simulink model "vdc_dyc_v3"  (R2020a)
settings: Solver=ode4  StartTime=0.0  StopTime=inf  FixedStep=1e-3  RelTol=1e-3
InitFcn:
  | clear mex
values from neighbouring files (symbols this model uses):
  vicrt_inputfile = append(path_send,              '2261_VOLCANO_ramp_RH12002_send_svm.xml')    [select_maneuver_files.m]
undefined symbols (not defined in the file or in its folder): vicrt_initcallback, vicrt_initmexcallback, vicrt_simulationmanager
libraries: simulink x1
(part 1 of 5)
settings Model: Creator=mcava  LastModifiedBy=lucas
settings DataIOCC: LimitDataPoints=on  SaveFormat=Array  ReturnWorkspaceOutputs=off  SignalLoggingName=sigsOut
settings OptimizationCC: ExpressionDepthLimit=2147483647  InitFltsAndDblsToZero=on  LifeSpan=inf
settings DebuggingCC: SignalInfNanChecking=warning  AlgebraicLoopMsg=none  SaveWithParameterizedLinksMsg=none  UnderspecifiedInitializationDetection=Classic  MergeDetectMultiDrivingBlocksExec=none  SignalResolutionControl=TryResolveAllWithWarning  MultiTaskDSMMsg=warning  MultiTaskCondExecSysMsg=none  FcnCallInpInsideContextMsg=warning  StateNameClashWarn=warning  SFUnexpectedBacktrackingDiag=warning  SFNoUnconditionalDefaultTransitionDiag=warning  SFExecutionAtInitializationDiag=none  ArithmeticOperatorsInVariantConditions=warning
settings HardwareCC: ProdBitPerPointer=32  ProdBitPerSizeT=32  ProdBitPerPtrDiffT=32  ProdLargestAtomicFloat=None  ProdIntDivRoundTo=Undefined  ProdEndianess=Unspecified  ProdWordSize=32  ProdHWDeviceType=32-bit Generic  TargetBitPerPointer=64  TargetBitPerSizeT=64  TargetBitPerPtrDiffT=64  TargetLongLongMode=on  TargetIntDivRoundTo=Zero  TargetEndianess=LittleEndian  TargetWordSize=64  TargetHWDeviceType=MATLAB Host  ProdEqTarget=off
settings ModelReferenceCC: PropagateSignalLabelsOutOfModel=off
settings SFSimCC: SimUseLocalCustomCode=off  SimParseCustomCode=off  CustomCodeUndefinedFunction=UseInterfaceOnly
settings RTWCC: RTWVerbose=off  RTWUseLocalCustomCode=off
settings CodeAppCC: GenerateComments=off  SimulinkBlockComments=off
settings GRTTargetCC: TargetFcnLib=ansi_tfl_tmw.mat  TargetLangStandard=C89/C90 (ANSI)  CombineOutputUpdateFcns=off  GRTInterface=on
settings ConfigComp: CovMetricSettings=dw  CovHtmlReporting=on  CovSaveCumulativeToWorkspaceVar=on  CovSaveSingleToWorkspaceVar=on  CovExternalEMLEnable=off

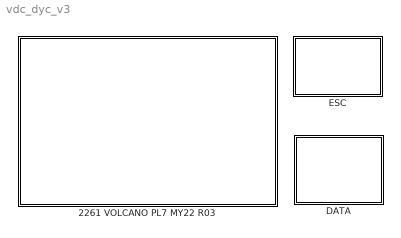
== system vdc_dyc_v3 ==
  2261 VOLCANO PL7 MY22 R03 : Subsystem
      mask Display: image(imread('C:\Users\lucas\Desktop\PPMEC_2023\Fiat_Toro.jpg'))
  DATA : Subsystem
      mask Display: image(imread('C:\Users\lucas\Desktop\PPMEC_2023\obd2.jpg'))
  ESC : Subsystem  mask(ESC Controller){ESCActive=on, WheelBase=2.989, vmass=1.344e3, wfront=548, wrear=796, FNOMIN=4.3e3, PKY1=-18.2127, PKY2=1.3905, PKY4=2, PPY1=0.4195, PPY2=1.2476, LKY=1}
      mask prompts: ESCActive "Active"; WheelBase "Wheel Base [m]"; vmass "Vehicle Mass [kg]"; wfront "Wiegth Front [kg]"; wrear "Wiegth Rear [kg]"
      mask help:
      | Enable/Disable ESC On/Off
      | Vehicle parameters are used  to calculate the Yaw Rate Target.
      mask DialogControl Container7 Prompt: Vehicle Settings
      mask DialogControl Container4 Prompt: Tyre Parameters
      mask DialogControl Control2 Prompt: Adjust accordingly to the tyre to be evaluated
      mask DialogControl Control3 Prompt: Fill in with the tyre(.tir) file parameters
      mask Display: image(imread('esp.jpg'))

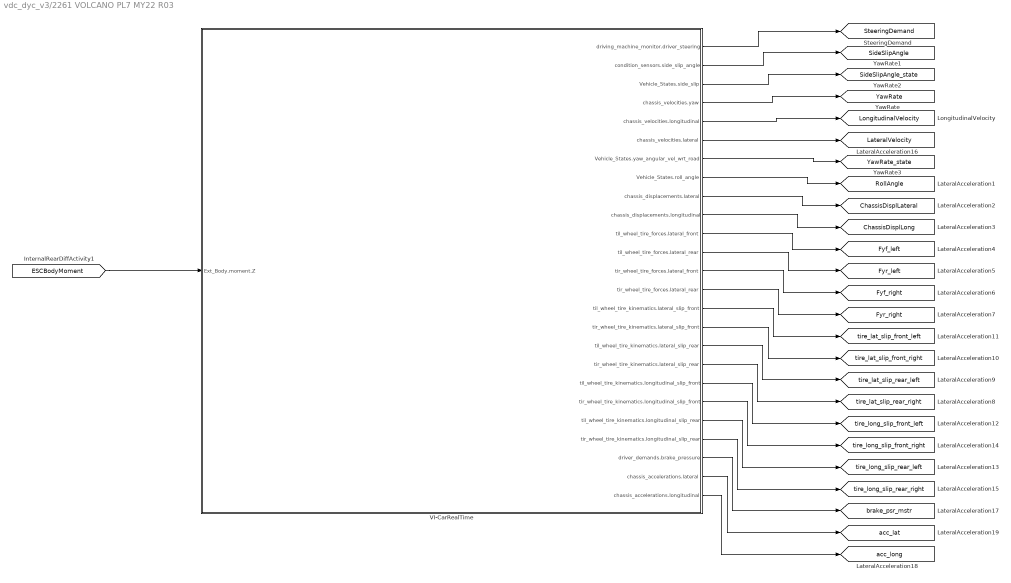
== system vdc_dyc_v3/2261 VOLCANO PL7 MY22 R03 ==
  VI-CarRealTime : Subsystem  InitFcn=vicrt_simulationmanager(0);  TreatAsAtomicUnit=on
      mask help: Full VI-CarRealTime mex integrated with IO Bus
      settings: CopyFcn=set_param(gcb, 'LinkStatus', 'none');  ModelCloseFcn=vicrt_simulationmanager(2);  OpenFcn=vicrt_simulationmanager(1);
      mask Display: image(imread('vehicle.jpg'));color('red');port_label('input',1,'Ext_Body.moment.Z');port_label('output',1,'driving_machine_monitor.driver_steering');port_label('output',2,'condition_sensors.side_slip_angle');port_label('output',3,'Vehicle_States.side_slip');port_label('output',4,'chassis_velocities.yaw');port_label('output',5,'chassis_velocities.longitudinal');port_label('output',6,'chassis_velocities.lateral');port_label('output',7,'Vehicle_States.yaw_angular_vel_wrt_road');port_label('output',8,'Vehicle_States.roll_angle');port_label('output',9,'chassis_displacements.lateral');port_label('output',10,'chassis_displacements.longitudinal');port_label('output',11,'til_wheel_tire_forces.lateral_front');port_label('output',12,'til_wheel_tire_forces.lateral_rear');port_label('output',13,'tir_wheel_tire_forces.lateral_front');port_label('output',14,'tir_wheel_tire_forces.lateral_rear');port_label('output',15,'til_wheel_tire_kinematics.lateral_slip_front');port_label('output',16,'tir_wheel_tire_kinematics.lateral_slip_front');port_label('output',17,'til_wheel_tire_kinematics.lateral_slip_rear');port_label('output',18,'tir_wheel_tire_kinematics.lateral_slip_rear');port_label('output',19,'til_wheel_tire_kinematics.longitudinal_slip_front');port_label('output',20,'tir_wheel_tire_kinematics.longitudinal_slip_front');port_label('output',21,'til_wheel_tire_kinematics.longitudinal_slip_rear');port_label('output',22,'tir_wheel_tire_kinematics.longitudinal_slip_rear');port_label('output',23,'driver_demands.brake_pressure');port_label('output',24,'chassis_accelerations.lateral');port_label('output',25,'chassis_accelerations.longitudinal');
  tag scope: ChassisDisplLateral=global, ChassisDisplLong=global, Fyf_left=global, Fyf_right=global, Fyr_left=global, Fyr_right=global, LateralVelocity=global, LongitudinalVelocity=global, RollAngle=global, SideSlipAngle=global, SideSlipAngle_state=global, SteeringDemand=global, YawRate=global, YawRate_state=global, acc_lat=global, acc_long=global, brake_psr_mstr=global, tire_lat_slip_front_left=global, tire_lat_slip_front_right=global, tire_lat_slip_rear_left=global, tire_lat_slip_rear_right=global, tire_long_slip_front_left=global, tire_long_slip_front_right=global, tire_long_slip_rear_left=global, tire_long_slip_rear_right=global
  wires:
  VI-CarRealTime/1(driving_machine_monitor.driver_steering) -> [SteeringDemand]
  VI-CarRealTime/4(chassis_velocities.yaw) -> [YawRate]
  VI-CarRealTime/5(chassis_velocities.longitudinal) -> [LongitudinalVelocity]
  [ESCBodyMoment] -> VI-CarRealTime/1(Ext_Body.moment.Z)
  VI-CarRealTime/8(Vehicle_States.roll_angle) -> [RollAngle]
  VI-CarRealTime/9(chassis_displacements.lateral) -> [ChassisDisplLateral]
  VI-CarRealTime/10(chassis_displacements.longitudinal) -> [ChassisDisplLong]
  VI-CarRealTime/11(til_wheel_tire_forces.lateral_front) -> [Fyf_left]
  VI-CarRealTime/12(til_wheel_tire_forces.lateral_rear) -> [Fyr_left]
  VI-CarRealTime/2(condition_sensors.side_slip_angle) -> [SideSlipAngle]
  VI-CarRealTime/14(tir_wheel_tire_forces.lateral_rear) -> [Fyr_right]
  VI-CarRealTime/13(tir_wheel_tire_forces.lateral_front) -> [Fyf_right]
  VI-CarRealTime/15(til_wheel_tire_kinematics.lateral_slip_front) -> [tire_lat_slip_front_left]
  VI-CarRealTime/16(tir_wheel_tire_kinematics.lateral_slip_front) -> [tire_lat_slip_front_right]
  VI-CarRealTime/17(til_wheel_tire_kinematics.lateral_slip_rear) -> [tire_lat_slip_rear_left]
  VI-CarRealTime/18(tir_wheel_tire_kinematics.lateral_slip_rear) -> [tire_lat_slip_rear_right]
  VI-CarRealTime/19(til_wheel_tire_kinematics.longitudinal_slip_front) -> [tire_long_slip_front_left]
  VI-CarRealTime/21(til_wheel_tire_kinematics.longitudinal_slip_rear) -> [tire_long_slip_rear_left]
  VI-CarRealTime/22(tir_wheel_tire_kinematics.longitudinal_slip_rear) -> [tire_long_slip_rear_right]
  VI-CarRealTime/20(tir_wheel_tire_kinematics.longitudinal_slip_front) -> [tire_long_slip_front_right]
  VI-CarRealTime/3(Vehicle_States.side_slip) -> [SideSlipAngle_state]
  VI-CarRealTime/7(Vehicle_States.yaw_angular_vel_wrt_road) -> [YawRate_state]
  VI-CarRealTime/6(chassis_velocities.lateral) -> [LateralVelocity]
  VI-CarRealTime/23(driver_demands.brake_pressure) -> [brake_psr_mstr]
  VI-CarRealTime/24(chassis_accelerations.lateral) -> [acc_lat]
  VI-CarRealTime/25(chassis_accelerations.longitudinal) -> [acc_long]

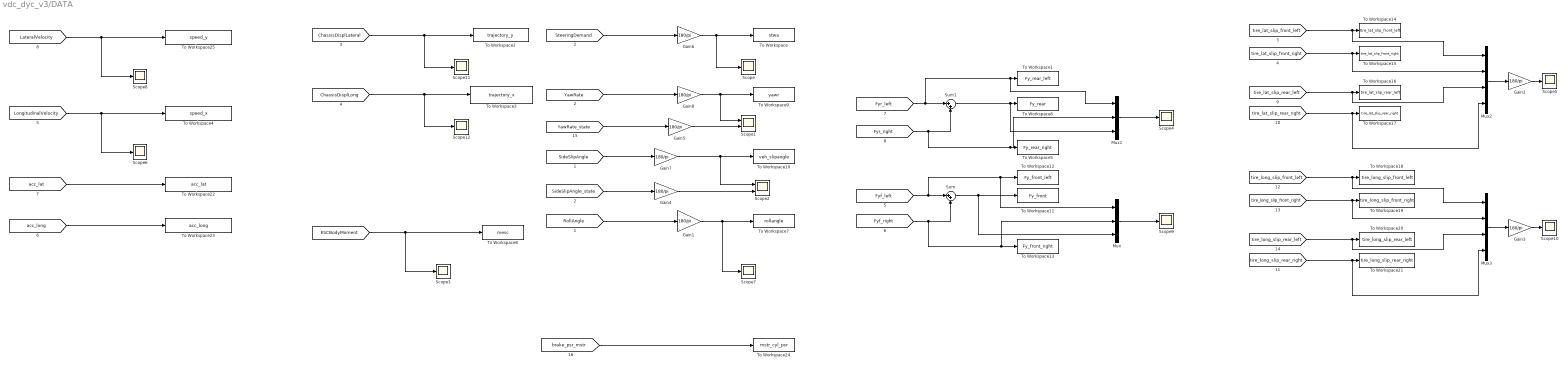
== system vdc_dyc_v3/DATA ==
  Gain{1..8} (8 alike) : Gain  Gain=180/pi
  Mux : Mux  Inputs=3
  Mux1 : Mux  Inputs=3
  Mux2 : Mux
  Mux3 : Mux
  Scope{,3..12} (11 alike) : Scope
  Scope1 : Scope  NumInputPorts=2
  Scope2 : Scope  NumInputPorts=2
  Sum : Sum  Inputs=|++
  Sum1 : Sum  Inputs=|++
  To Workspace : ToWorkspace  VariableName=stwa  SaveFormat=Timeseries  SampleTime=-1
  To Workspace1 : ToWorkspace  VariableName=Fy_rear_left  SaveFormat=Timeseries  SampleTime=-1
  To Workspace10 : ToWorkspace  VariableName=veh_slipangle  SaveFormat=Timeseries  SampleTime=-1
  To Workspace11 : ToWorkspace  VariableName=Fy_front  SaveFormat=Timeseries  SampleTime=-1
  To Workspace12 : ToWorkspace  VariableName=Fy_front_left  SaveFormat=Timeseries  SampleTime=-1
  To Workspace13 : ToWorkspace  VariableName=Fy_front_right  SaveFormat=Timeseries  SampleTime=-1
  To Workspace14 : ToWorkspace  VariableName=tire_lat_slip_front_left  SaveFormat=Timeseries  SampleTime=-1
  To Workspace15 : ToWorkspace  VariableName=tire_lat_slip_front_right  SaveFormat=Timeseries  SampleTime=-1
  To Workspace16 : ToWorkspace  VariableName=tire_lat_slip_rear_left  SaveFormat=Timeseries  SampleTime=-1
  To Workspace17 : ToWorkspace  VariableName=tire_lat_slip_rear_right  SaveFormat=Timeseries  SampleTime=-1
  To Workspace18 : ToWorkspace  VariableName=tire_long_slip_front_left  SaveFormat=Timeseries  SampleTime=-1
  To Workspace19 : ToWorkspace  VariableName=tire_long_slip_front_right  SaveFormat=Timeseries  SampleTime=-1
  To Workspace2 : ToWorkspace  VariableName=trajectory_y  SaveFormat=Timeseries  SampleTime=-1
  To Workspace20 : ToWorkspace  VariableName=tire_long_slip_rear_left  SaveFormat=Timeseries  SampleTime=-1
  To Workspace21 : ToWorkspace  VariableName=tire_long_slip_rear_right  SaveFormat=Timeseries  SampleTime=-1
  To Workspace22 : ToWorkspace  VariableName=acc_lat  SaveFormat=Timeseries  SampleTime=-1
  To Workspace23 : ToWorkspace  VariableName=acc_long  SaveFormat=Timeseries  SampleTime=-1
  To Workspace24 : ToWorkspace  VariableName=mstr_cyl_psr  SaveFormat=Timeseries  SampleTime=-1
  To Workspace25 : ToWorkspace  VariableName=speed_y  SaveFormat=Timeseries  SampleTime=-1
  To Workspace3 : ToWorkspace  VariableName=trajectory_x  SaveFormat=Timeseries  SampleTime=-1
  To Workspace4 : ToWorkspace  VariableName=speed_x  SaveFormat=Timeseries  SampleTime=-1
  To Workspace5 : ToWorkspace  VariableName=Fy_rear_right  SaveFormat=Timeseries  SampleTime=-1
  To Workspace6 : ToWorkspace  VariableName=Fy_rear  SaveFormat=Timeseries  SampleTime=-1
  To Workspace7 : ToWorkspace  VariableName=rollangle  SaveFormat=Timeseries  SampleTime=-1
  To Workspace8 : ToWorkspace  VariableName=mesc  SaveFormat=Timeseries  SampleTime=-1
  To Workspace9 : ToWorkspace  VariableName=yawr  SaveFormat=Timeseries  SampleTime=-1
  wires:
  [LongitudinalVelocity] -> Scope6/1, To Workspace4/1
  [RollAngle] -> Gain1/1
  [ESCBodyMoment] -> Scope3/1, To Workspace8/1
  Gain1/1 -> To Workspace7/1, Scope7/1
  [SteeringDemand] -> Gain6/1
  Gain6/1 -> To Workspace/1, Scope/1
  Gain7/1 -> To Workspace10/1, Scope2/1
  Gain8/1 -> To Workspace9/1, Scope1/1
  [SideSlipAngle] -> Gain7/1
  [ChassisDisplLong] -> To Workspace3/1, Scope12/1
  [YawRate] -> Gain8/1
  [ChassisDisplLateral] -> To Workspace2/1, Scope11/1
  [Fyf_left] -> Sum/1, Mux/1, To Workspace12/1
  Sum/1 -> Mux/3, To Workspace11/1
  [Fyr_left] -> Mux1/1, To Workspace1/1, Sum1/1
  [Fyr_right] -> Mux1/2, To Workspace5/1, Sum1/2
  Sum1/1 -> Mux1/3, To Workspace6/1
  [Fyf_right] -> Mux/2, To Workspace13/1, Sum/2
  Mux/1 -> Scope9/1
  Mux1/1 -> Scope4/1
  [tire_lat_slip_front_left] -> Mux2/1, To Workspace14/1
  [tire_lat_slip_front_right] -> Mux2/2, To Workspace15/1
  [tire_lat_slip_rear_left] -> Mux2/3, To Workspace16/1
  [tire_lat_slip_rear_right] -> Mux2/4, To Workspace17/1
  Mux2/1 -> Gain2/1
  Gain2/1 -> Scope5/1
  Mux3/1 -> Gain3/1
  [tire_long_slip_rear_right] -> Mux3/4, To Workspace21/1
  Gain3/1 -> Scope10/1
  [tire_long_slip_rear_left] -> Mux3/3, To Workspace20/1
  [tire_long_slip_front_left] -> Mux3/1, To Workspace18/1
  [tire_long_slip_front_right] -> Mux3/2, To Workspace19/1
  [SideSlipAngle_state] -> Gain4/1
  Gain4/1 -> Scope2/2
  Gain5/1 -> Scope1/2
  [YawRate_state] -> Gain5/1
  [acc_long] -> To Workspace23/1
  [acc_lat] -> To Workspace22/1
  [brake_psr_mstr] -> To Workspace24/1
  [LateralVelocity] -> Scope8/1, To Workspace25/1

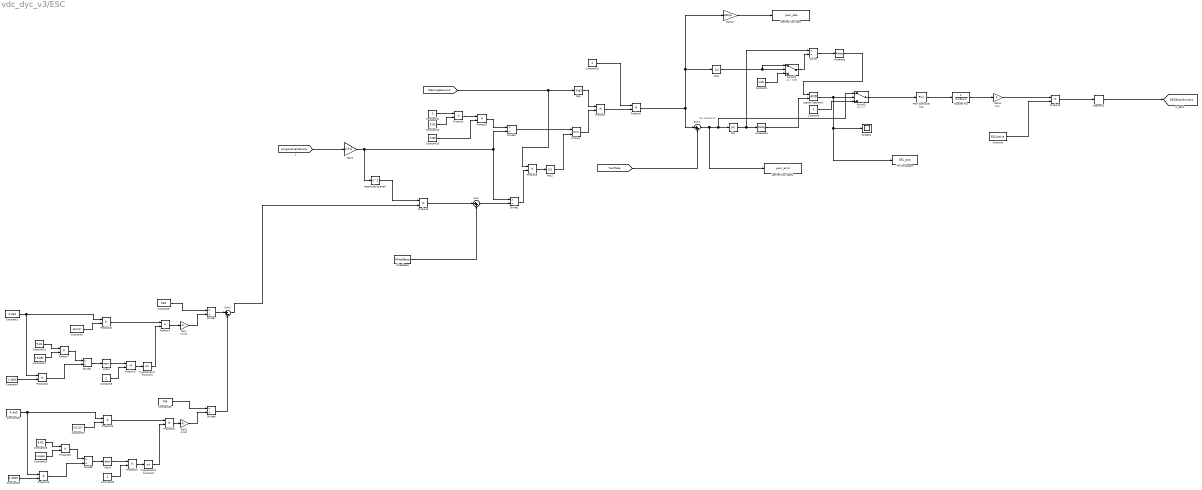
== system vdc_dyc_v3/ESC ==
  note: Gain
  note: Yaw Rate Error
  "\"PID\" Controller Yaw" : simulink/Continuous/PID Controller  Controller=P  Form=Parallel  TimeDomain=Continuous-time  UseExternalTs=off  SampleTime=-1  IntegratorMethod=Forward Euler  FilterMethod=Forward Euler  ControllerParametersSource=internal  P=9.9912e4  I=0  D=1e7  UseFilter=on  N=1e-3  TunerSelectOption=Frequency Response Based  InitialConditionSource=internal  InitialConditionForIntegrator=0  InitialConditionForFilter=0  DifferentiatorICPrevScaledInput=0  ExternalReset=none  TrackingMode=off  Kt=1  LimitOutput=off  UpperSaturationLimit=inf  LowerSaturationLimit=-inf  LinearizeAsGain=on  AntiWindupMode=none  Kb=1  POutMin=[]  POutMax=[]  IOutMin=[]  IOutMax=[]  DOutMin=[]  DOutMax=[]  NOutMin=[]  NOutMax=[]  SumOutMin=[]  SumOutMax=[]  SaturationOutMin=[]  SaturationOutMax=[]  PParamMin=[]  PParamMax=[]  IParamMin=[]  IParamMax=[]  DParamMin=[]  DParamMax=[]  NParamMin=[]  NParamMax=[]  KbParamMin=[]  KbParamMax=[]  KtParamMin=[]  KtParamMax=[]  KbOutMin=[]  KbOutMax=[]  KtOutMin=[]  KtOutMax=[]  IntegratorOutMin=[]  IntegratorOutMax=[]  FilterOutMin=[]  FilterOutMax=[]  SumI1OutMin=[]  SumI1OutMax=[]  SumI2OutMin=[]  SumI2OutMax=[]  SumI3OutMin=[]  SumI3OutMax=[]  SumI4OutMin=[]  SumI4OutMax=[]  SumDOutMin=[]  SumDOutMax=[]  DifferentiatorOutMin=[]  DifferentiatorOutMax=[]  FilterDiffOutCoefMin=[]  FilterDiffOutCoefMax=[]  ReciprocalOutMin=[]  ReciprocalOutMax=[]  SumDenOutMin=[]  SumDenOutMax=[]  SumNumOutMin=[]  SumNumOutMax=[]  DivideOutMin=[]  DivideOutMax=[]  UdiffTsProdOutMin=[]  UdiffTsProdOutMax=[]  NTsProdOutMin=[]  NTsProdOutMax=[]  UintegralTsProdOutMin=[]  UintegralTsProdOutMax=[]  UngainTsProdOutMin=[]  UngainTsProdOutMax=[]  IntegratorContinuousStateAttributes=''  IntegratorStateMustResolveToSignalObject=off  IntegratorRTWStateStorageClass=Auto  FilterContinuousStateAttributes=''  FilterStateMustResolveToSignalObject=off  FilterRTWStateStorageClass=Auto  ParallelPVariant=InternalParameters  IdealPVariant=Disabled  IVariant=Disabled  DVariant=Disabled  IntegratorVariant=Disabled  SatVariant=Disabled  AWVariant=Disabled  PCopyVariant=Disabled  TRVariant=Disabled  FdbkBlocksVariant=Forward  IdealPFdbkVariant=Disabled  SatFdbkVariant=Disabled  DerivativeFilterVariant=Disabled  NVariant=Disabled  NCopyVariant=Disabled_SignalSpec  FilterICVariant=Disabled  IntegratorICVariant=Disabled  ExternalResetVariant=Disabled  TRSumVariant=Passthrough  SumFdbkVariant=Disabled  SumVariant=Passthrough_P  TsampFilterVariant=InternalTs  TsampNgainVariant=Passthrough  TsampIntegralVariant=Disabled_SignalSpec
  Abs : Abs
  Abs1 : Abs
  Abs2 : Abs
  Atan1 : Trigonometry  Operator=atan
  Atan2 : Trigonometry  Operator=atan
  Constant : Constant  Value=ESCActive
  Constant1 : Constant  Value=0.001
  Constant10 : Constant  Value=0.85
  Constant11 : Constant  Value=1.344e3
  Constant12 : Constant
  Constant13 : Constant  Value=9.81
  Constant15 : Constant
  Constant2 : Constant  Value=4.3e3
  Constant21 : Constant  Value=9.81
  Constant24 : Constant  Value=1.344e3
  Constant25 : Constant  Value=4.3e3
  Constant26 : Constant  Value=9.81
  Constant27 : Constant  Value=-18.2127
  Constant28 : Constant  Value=1.3905
  Constant29 : Constant  Value=2
  Constant3 : Constant  Value=-18.2127
  Constant30 : Constant  Value=796
  Constant4 : Constant  Value=1.3905
  Constant5 : Constant  Value=0
  Constant8 : Constant  Value=2
  Constant9 : Constant  Value=548
  Desired Yaw Rate : ToWorkspace  VariableName=yawr_des  SaveFormat=Timeseries  SampleTime=-1
  Desired Yaw Rate1 : ToWorkspace  VariableName=yawr_error  SaveFormat=Timeseries  SampleTime=-1
  Divide{,1..2,4,6..8} (7 alike) : Product  Inputs=*/
  Gain : Gain  Gain=pi/180
  Gain1 : Gain  Gain=pi/180
  Gain10 : Gain  Gain=180/pi
  Gain2 : Gain  Gain=1/3.6
  Gain3 : Gain
  Histerese : Relay  OnSwitchValue=0.02  OffSwitchValue=0
  Histerese1 : Relay  OnSwitchValue=0.15  OffSwitchValue=1e-4
  Logical Operator2 : Logic  AllPortsSameDT=off  OutDataTypeStr=boolean
  Magnitude Squared : Math  Operator=square  SaturateOnIntegerOverflow=on
  Memory1 : Memory
  MinMax : MinMax  Inputs=2
  Product{1..9,16..17,19..21,23..25} (17 alike) : Product  SaturateOnIntegerOverflow=on
  Scope21 : Scope
  Sign : Signum
  Sum : Sum  Inputs=|++
  Sum1 : Sum  Inputs=|+-
  Sum2 : Sum  Inputs=|+-
  Switch1 : Switch  Criteria=u2 > Threshold  ZeroCross=off
  Switch3 : Switch  Criteria=u2 > Threshold  Threshold=0.05  ZeroCross=off
  To Workspace : ToWorkspace  VariableName=ESC_actv  SaveFormat=Timeseries  SampleTime=-1
  Transfer Fcn : TransferFcn  Denominator=[0.15 1]
  Trigonometric Function1 : Trigonometry
  Trigonometric Function2 : Trigonometry
  WheelBase : Constant  Value=WheelBase
  tag scope: ESCBodyMoment=global
  wires:
  Gain10/1 -> Desired Yaw Rate/1
  MinMax/1 -> Product1/2
  Sign/1 -> Product1/1
  Logical Operator2/1 -> Switch1/2, To Workspace/1, Scope21/1
  Histerese1/1 -> Logical Operator2/2
  Constant5/1 -> Switch1/3
  Histerese/1 -> Logical Operator2/1
  Sum1/1 -> Desired Yaw Rate1/1, Switch1/1, Abs/1
  Switch3/1 -> Divide/2
  Product9/1 -> Memory1/1
  Gain3/1 -> Product9/1
  Constant/1 -> Product9/2
  Constant12/1 -> Product2/1
  Constant13/1 -> Product2/2
  [LongitudinalVelocity] -> Gain2/1
  Divide2/1 -> Product3/2
  Gain2/1 -> Divide2/1, Divide1/2, Magnitude Squared/1
  Abs1/1 -> Switch3/2, Switch3/1
  Memory1/1 -> [ESCBodyMoment]
  Divide/1 -> Histerese/1
  [SteeringDemand] -> Product3/1, Sign/1
  Product5/1 -> Divide1/1
  Product2/1 -> Product5/1
  Constant10/1 -> Product5/2
  Product3/1 -> Abs2/1
  Abs2/1 -> MinMax/2
  Divide1/1 -> MinMax/1
  Magnitude Squared/1 -> Product6/1
  WheelBase/1 -> Sum/2
  Sum/1 -> Divide2/2
  Constant1/1 -> Switch3/3
  [YawRate] -> Sum1/2
  Abs/1 -> Histerese1/1, Divide/1
  Constant15/1 -> Product8/1
  Switch1/1 -> "\"PID\" Controller Yaw"/1
  "\"PID\" Controller Yaw"/1 -> Transfer Fcn/1
  Product1/1 -> Product8/2
  Product6/1 -> Sum/1
  Transfer Fcn/1 -> Gain3/1
  Sum2/1 -> Product6/2
  Product8/1 -> Sum1/1, Gain10/1, Abs1/1
  Divide7/1 -> Sum2/1
  Constant8/1 -> Product17/2
  Atan1/1 -> Product17/1
  Product20/1 -> Product4/1
  Product16/1 -> Divide4/2
  Constant3/1 -> Product20/2
  Product7/1 -> Divide4/1
  Constant4/1 -> Product16/2
  Constant9/1 -> Divide7/1
  Trigonometric Function1/1 -> Product4/2
  Constant11/1 -> Product7/2
  Divide4/1 -> Atan1/1
  Constant21/1 -> Product7/1
  Product4/1 -> Gain/1
  Product17/1 -> Trigonometric Function1/1
  Constant2/1 -> Product20/1, Product16/1
  Divide8/1 -> Sum2/2
  Constant25/1 -> Product23/1, Product19/1
  Product21/1 -> Trigonometric Function2/1
  Product24/1 -> Gain1/1
  Divide6/1 -> Atan2/1
  Constant26/1 -> Product25/1
  Constant24/1 -> Product25/2
  Constant27/1 -> Product23/2
  Product23/1 -> Product24/1
  Product19/1 -> Divide6/2
  Constant28/1 -> Product19/2
  Atan2/1 -> Product21/1
  Constant29/1 -> Product21/2
  Product25/1 -> Divide6/1
  Constant30/1 -> Divide8/1
  Trigonometric Function2/1 -> Product24/2
  Gain/1 -> Divide7/2
  Gain1/1 -> Divide8/2

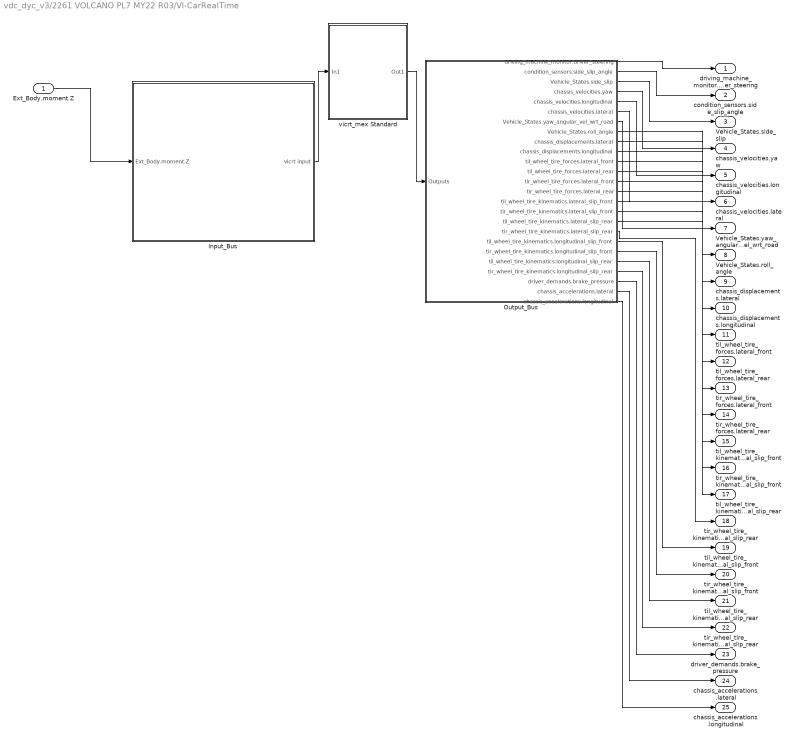
== system vdc_dyc_v3/2261 VOLCANO PL7 MY22 R03/VI-CarRealTime ==
  Ext_Body.moment.Z : Inport
  Input_Bus : Subsystem  LoadFcn=vicrt_initcallback(gcb)
      settings: CopyFcn=vicrt_initcallback(gcb)
  Output_Bus : Subsystem  Description=Outputs
      settings: CopyFcn=set_param(gcb, 'LinkStatus', 'none')
  vicrt_mex Standard : Subsystem  mask{vicrt_inputfile=vicrt_inputfile, vicrt_outprefix='', intStep=0.001, AniFlag=off, inpPortDim=389, outPortDim=1378, NoDirectFeedthrough=on}
      mask prompts: vicrt_inputfile "VI-CarRealtime input file"; vicrt_outprefix "VI-CarRealTime output prefix"; intStep "Integration step"; AniFlag "live animation"; inpPortDim "input port dimension"; outPortDim "output port dimension"; NoDirectFeedthrough "Direct Feedthrough Off"
      mask init:
      | custDriv=[1,1,1];
      settings: CopyFcn=set_param(gcb, 'LinkStatus', 'none')
  driving_machine_monitor.driver_steering : Outport
  condition_sensors.side_slip_angle : Outport  Port=2  VectorParamsAs1DForOutWhenUnconnected=off
  Vehicle_States.side_slip : Outport  Port=3
  chassis_velocities.yaw : Outport  Port=4  VectorParamsAs1DForOutWhenUnconnected=off
  chassis_velocities.longitudinal : Outport  Port=5
  chassis_velocities.lateral : Outport  Port=6
  Vehicle_States.yaw_angular_vel_wrt_road : Outport  Port=7
  Vehicle_States.roll_angle : Outport  Port=8
  chassis_displacements.lateral : Outport  Port=9
  chassis_displacements.longitudinal : Outport  Port=10
  til_wheel_tire_forces.lateral_front : Outport  Port=11
  til_wheel_tire_forces.lateral_rear : Outport  Port=12
  tir_wheel_tire_forces.lateral_front : Outport  Port=13
  tir_wheel_tire_forces.lateral_rear : Outport  Port=14
  til_wheel_tire_kinematics.lateral_slip_front : Outport  Port=15
  tir_wheel_tire_kinematics.lateral_slip_front : Outport  Port=16
  til_wheel_tire_kinematics.lateral_slip_rear : Outport  Port=17
  tir_wheel_tire_kinematics.lateral_slip_rear : Outport  Port=18
  til_wheel_tire_kinematics.longitudinal_slip_front : Outport  Port=19
  tir_wheel_tire_kinematics.longitudinal_slip_front : Outport  Port=20
  til_wheel_tire_kinematics.longitudinal_slip_rear : Outport  Port=21
  tir_wheel_tire_kinematics.longitudinal_slip_rear : Outport  Port=22
  driver_demands.brake_pressure : Outport  Port=23
  chassis_accelerations.lateral : Outport  Port=24
  chassis_accelerations.longitudinal : Outport  Port=25
  wires:
  vicrt_mex Standard/1(Out1) -> Output_Bus/1(Outputs)
  Input_Bus/1(vicrt input) -> vicrt_mex Standard/1(In1)
  Ext_Body.moment.Z/1 -> Input_Bus/1(Ext_Body.moment.Z)
  Output_Bus/1(driving_machine_monitor.driver_steering) -> driving_machine_monitor.driver_steering/1
  Output_Bus/2(condition_sensors.side_slip_angle) -> condition_sensors.side_slip_angle/1
  Output_Bus/3(Vehicle_States.side_slip) -> Vehicle_States.side_slip/1
  Output_Bus/4(chassis_velocities.yaw) -> chassis_velocities.yaw/1
  Output_Bus/5(chassis_velocities.longitudinal) -> chassis_velocities.longitudinal/1
  Output_Bus/6(chassis_velocities.lateral) -> chassis_velocities.lateral/1
  Output_Bus/7(Vehicle_States.yaw_angular_vel_wrt_road) -> Vehicle_States.yaw_angular_vel_wrt_road/1
  Output_Bus/8(Vehicle_States.roll_angle) -> Vehicle_States.roll_angle/1
  Output_Bus/9(chassis_displacements.lateral) -> chassis_displacements.lateral/1
  Output_Bus/10(chassis_displacements.longitudinal) -> chassis_displacements.longitudinal/1
  Output_Bus/11(til_wheel_tire_forces.lateral_front) -> til_wheel_tire_forces.lateral_front/1
  Output_Bus/12(til_wheel_tire_forces.lateral_rear) -> til_wheel_tire_forces.lateral_rear/1
  Output_Bus/13(tir_wheel_tire_forces.lateral_front) -> tir_wheel_tire_forces.lateral_front/1
  Output_Bus/14(tir_wheel_tire_forces.lateral_rear) -> tir_wheel_tire_forces.lateral_rear/1
  Output_Bus/15(til_wheel_tire_kinematics.lateral_slip_front) -> til_wheel_tire_kinematics.lateral_slip_front/1
  Output_Bus/16(tir_wheel_tire_kinematics.lateral_slip_front) -> tir_wheel_tire_kinematics.lateral_slip_front/1
  Output_Bus/17(til_wheel_tire_kinematics.lateral_slip_rear) -> til_wheel_tire_kinematics.lateral_slip_rear/1
  Output_Bus/18(tir_wheel_tire_kinematics.lateral_slip_rear) -> tir_wheel_tire_kinematics.lateral_slip_rear/1
  Output_Bus/19(til_wheel_tire_kinematics.longitudinal_slip_front) -> til_wheel_tire_kinematics.longitudinal_slip_front/1
  Output_Bus/20(tir_wheel_tire_kinematics.longitudinal_slip_front) -> tir_wheel_tire_kinematics.longitudinal_slip_front/1
  Output_Bus/21(til_wheel_tire_kinematics.longitudinal_slip_rear) -> til_wheel_tire_kinematics.longitudinal_slip_rear/1
  Output_Bus/22(tir_wheel_tire_kinematics.longitudinal_slip_rear) -> tir_wheel_tire_kinematics.longitudinal_slip_rear/1
  Output_Bus/23(driver_demands.brake_pressure) -> driver_demands.brake_pressure/1
  Output_Bus/24(chassis_accelerations.lateral) -> chassis_accelerations.lateral/1
  Output_Bus/25(chassis_accelerations.longitudinal) -> chassis_accelerations.longitudinal/1

== system vdc_dyc_v3/2261 VOLCANO PL7 MY22 R03/VI-CarRealTime/Input_Bus ==
  Ext_Body.moment.Z : Inport
  Bus2Map : Subsystem
  Inputs : Subsystem
  VicrtBusAssignment : BusAssignment  AssignedSignals=Ext_Body.moment.Z
  vicrt input : Outport  VectorParamsAs1DForOutWhenUnconnected=off
  wires:
  Bus2Map/1(Map Out) -> vicrt input/1
  VicrtBusAssignment/1 -> Bus2Map/1(Bus In)
  Inputs/1(Inputs) -> VicrtBusAssignment/1  "Inputs"
  Ext_Body.moment.Z/1 -> VicrtBusAssignment/2

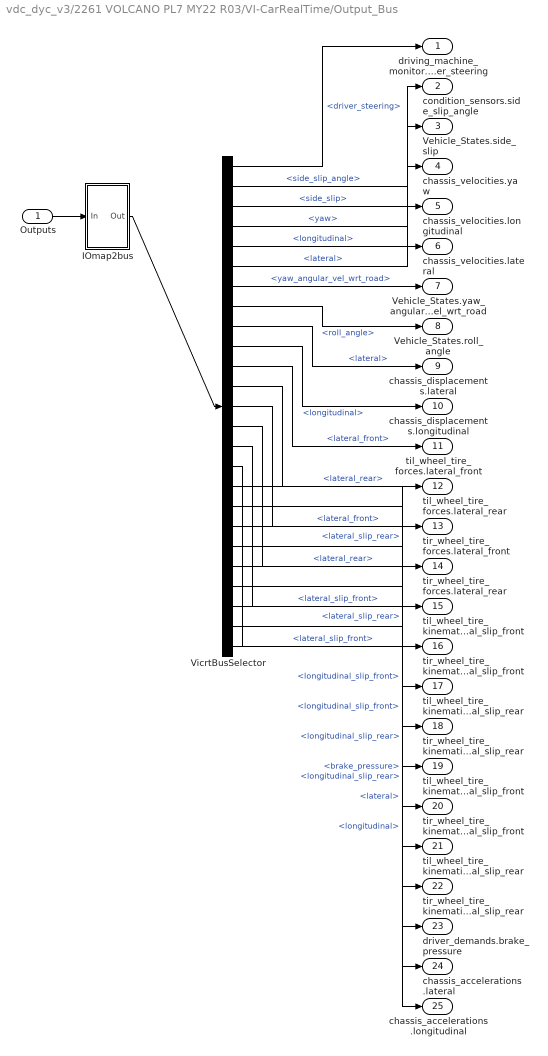
== system vdc_dyc_v3/2261 VOLCANO PL7 MY22 R03/VI-CarRealTime/Output_Bus ==
  Outputs : Inport
  IOmap2bus : Subsystem
  VicrtBusSelector : BusSelector  OutputSignals=driving_machine_monitor.driver_steering,condition_sensors.side_slip_angle,Vehicle_States.side_slip,chassis_velocities.yaw,chassis_velocities.longitudinal,chassis_velocities.lateral,Vehicle_States.yaw_angular_vel_wrt_road,Vehicle_States.roll_angle,chassis_displacements.lateral,chassis_displacements.longitudinal,til_wheel_tire_forces.lateral_front,til_wheel_tire_forces.lateral_rear,tir_wheel_tire_forces.lateral_front,tir_wheel_tire_forces.lateral_rear,til_wheel_tire_kinematics.lateral_slip_front,tir_wheel_tire_kinematics.lateral_slip_front,til_wheel_tire_kinematics.lateral_slip_rear,tir_wheel_tire_kinematics.lateral_slip_rear,til_wheel_tire_kinematics.longitudinal_slip_front,tir_wheel_tire_kinematics.longitudinal_slip_front,til_wheel_tire_kinematics.longitudinal_slip_rear,tir_wheel_tire_kinematics.longitudinal_slip_rear,driver_demands.brake_pressure,chassis_accelerations.lateral,chassis_accelerations.longitudinal
  driving_machine_monitor.driver_steering : Outport
  condition_sensors.side_slip_angle : Outport  Port=2  VectorParamsAs1DForOutWhenUnconnected=off
  Vehicle_States.side_slip : Outport  Port=3
  chassis_velocities.yaw : Outport  Port=4  VectorParamsAs1DForOutWhenUnconnected=off
  chassis_velocities.longitudinal : Outport  Port=5
  chassis_velocities.lateral : Outport  Port=6
  Vehicle_States.yaw_angular_vel_wrt_road : Outport  Port=7
  Vehicle_States.roll_angle : Outport  Port=8
  chassis_displacements.lateral : Outport  Port=9
  chassis_displacements.longitudinal : Outport  Port=10
  til_wheel_tire_forces.lateral_front : Outport  Port=11
  til_wheel_tire_forces.lateral_rear : Outport  Port=12
  tir_wheel_tire_forces.lateral_front : Outport  Port=13
  tir_wheel_tire_forces.lateral_rear : Outport  Port=14
  til_wheel_tire_kinematics.lateral_slip_front : Outport  Port=15
  tir_wheel_tire_kinematics.lateral_slip_front : Outport  Port=16
  til_wheel_tire_kinematics.lateral_slip_rear : Outport  Port=17
  tir_wheel_tire_kinematics.lateral_slip_rear : Outport  Port=18
  til_wheel_tire_kinematics.longitudinal_slip_front : Outport  Port=19
  tir_wheel_tire_kinematics.longitudinal_slip_front : Outport  Port=20
  til_wheel_tire_kinematics.longitudinal_slip_rear : Outport  Port=21
  tir_wheel_tire_kinematics.longitudinal_slip_rear : Outport  Port=22
  driver_demands.brake_pressure : Outport  Port=23
  chassis_accelerations.lateral : Outport  Port=24
  chassis_accelerations.longitudinal : Outport  Port=25
  wires:
  IOmap2bus/1(Out) -> VicrtBusSelector/1
  Outputs/1 -> IOmap2bus/1(In)
  VicrtBusSelector/1 -> driving_machine_monitor.driver_steering/1  "<driver_steering>"
  VicrtBusSelector/2 -> condition_sensors.side_slip_angle/1  "<side_slip_angle>"
  VicrtBusSelector/3 -> Vehicle_States.side_slip/1  "<side_slip>"
  VicrtBusSelector/4 -> chassis_velocities.yaw/1  "<yaw>"
  VicrtBusSelector/5 -> chassis_velocities.longitudinal/1  "<longitudinal>"
  VicrtBusSelector/6 -> chassis_velocities.lateral/1  "<lateral>"
  VicrtBusSelector/7 -> Vehicle_States.yaw_angular_vel_wrt_road/1  "<yaw_angular_vel_wrt_road>"
  VicrtBusSelector/8 -> Vehicle_States.roll_angle/1  "<roll_angle>"
  VicrtBusSelector/9 -> chassis_displacements.lateral/1  "<lateral>"
  VicrtBusSelector/10 -> chassis_displacements.longitudinal/1  "<longitudinal>"
  VicrtBusSelector/11 -> til_wheel_tire_forces.lateral_front/1  "<lateral_front>"
  VicrtBusSelector/12 -> til_wheel_tire_forces.lateral_rear/1  "<lateral_rear>"
  VicrtBusSelector/13 -> tir_wheel_tire_forces.lateral_front/1  "<lateral_front>"
  VicrtBusSelector/14 -> tir_wheel_tire_forces.lateral_rear/1  "<lateral_rear>"
  VicrtBusSelector/15 -> til_wheel_tire_kinematics.lateral_slip_front/1  "<lateral_slip_front>"
  VicrtBusSelector/16 -> tir_wheel_tire_kinematics.lateral_slip_front/1  "<lateral_slip_front>"
  VicrtBusSelector/17 -> til_wheel_tire_kinematics.lateral_slip_rear/1  "<lateral_slip_rear>"
  VicrtBusSelector/18 -> tir_wheel_tire_kinematics.lateral_slip_rear/1  "<lateral_slip_rear>"
  VicrtBusSelector/19 -> til_wheel_tire_kinematics.longitudinal_slip_front/1  "<longitudinal_slip_front>"
  VicrtBusSelector/20 -> tir_wheel_tire_kinematics.longitudinal_slip_front/1  "<longitudinal_slip_front>"
  VicrtBusSelector/21 -> til_wheel_tire_kinematics.longitudinal_slip_rear/1  "<longitudinal_slip_rear>"
  VicrtBusSelector/22 -> tir_wheel_tire_kinematics.longitudinal_slip_rear/1  "<longitudinal_slip_rear>"
  VicrtBusSelector/23 -> driver_demands.brake_pressure/1  "<brake_pressure>"
  VicrtBusSelector/24 -> chassis_accelerations.lateral/1  "<lateral>"
  VicrtBusSelector/25 -> chassis_accelerations.longitudinal/1  "<longitudinal>"

== system vdc_dyc_v3/2261 VOLCANO PL7 MY22 R03/VI-CarRealTime/vicrt_mex Standard ==
  In1 : Inport
  vicrt_mex : S-Function  InitFcn=vicrt_initmexcallback(gcb);  FunctionName=vicrt_mex  Parameters=vicrt_inputfile,vicrt_outprefix,AniFlag,intStep,inpPortDim,outPortDim,NoDirectFeedthrough  SFunctionDeploymentMode=off  EnableBusSupport=off
  Out1 : Outport  VectorParamsAs1DForOutWhenUnconnected=off
  wires:
  In1/1 -> vicrt_mex/1
  vicrt_mex/1 -> Out1/1
